simulink model "gm_tutorial1_1_vnl"  (R2020b)
settings: Solver=FixedStepDiscrete  StartTime=0.0  StopTime=simulation_stop_time  RelTol=1e-3
undefined symbols (not defined in the file or in its folder): sample_time
libraries: simulink x3
settings Model: Creator=yixingli  LastModifiedBy=harsh
settings DataIOCC: LimitDataPoints=on  SaveOutput=off  SignalLogging=off  SaveTime=off
settings OptimizationCC: BlockReduction=off  ConditionallyExecuteInputs=off  DefaultParameterBehavior=Inlined  ExpressionDepthLimit=2147483647  LifeSpan=inf
settings DebuggingCC: AlgebraicLoopMsg=error  UnderspecifiedInitializationDetection=Classic  MergeDetectMultiDrivingBlocksExec=none  InheritedTsInSrcMsg=none  SingleTaskRateTransMsg=error  ParameterPrecisionLossMsg=none  AllowSymbolicDim=off  StateNameClashWarn=warning  StrictBusMsg=ErrorOnBusTreatedAsVector  SFUnexpectedBacktrackingDiag=warning  SFNoUnconditionalDefaultTransitionDiag=warning  SFExecutionAtInitializationDiag=none  ArithmeticOperatorsInVariantConditions=warning
settings HardwareCC: ProdBitPerPointer=32  ProdBitPerSizeT=32  ProdBitPerPtrDiffT=32  ProdLargestAtomicFloat=None  ProdIntDivRoundTo=Undefined  ProdEndianess=Unspecified  ProdWordSize=32  ProdHWDeviceType=ASIC/FPGA->ASIC/FPGA  ProdEqTarget=off
settings SFSimCC: SimUseLocalCustomCode=off  CustomCodeUndefinedFunction=UseInterfaceOnly
settings RTWCC: RTWUseLocalCustomCode=off
settings CodeAppCC: StateflowObjectComments=on
settings GRTTargetCC: TargetLangStandard=C89/C90 (ANSI)
settings ConfigComp: CovScope=ReferencedModels  CovMetricSettings=dw  CovSaveCumulativeToWorkspaceVar=on  CovSaveSingleToWorkspaceVar=on  CovExternalEMLEnable=off  CovSFcnEnable=off

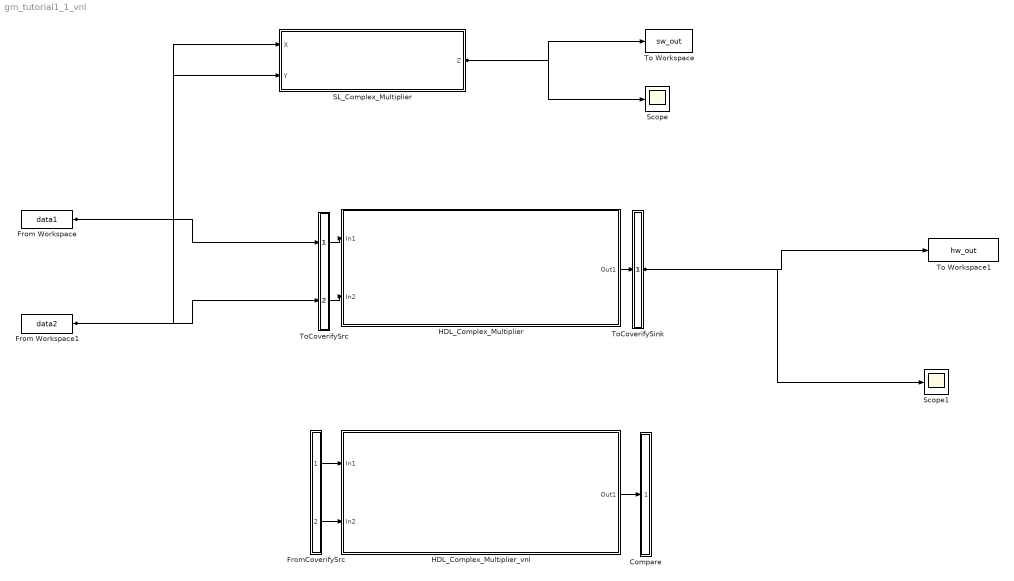
== system gm_tutorial1_1_vnl ==
  Compare : Subsystem
      mask Display: disp('')
  From Workspace : FromWorkspace  VariableName=data1  SampleTime=sample_time  Interpolate=off  OutputAfterFinalValue=Setting to zero
  From Workspace1 : FromWorkspace  VariableName=data2  SampleTime=sample_time  Interpolate=off  OutputAfterFinalValue=Setting to zero
  FromCoverifySrc : Subsystem
      mask Display: disp('')
  HDL_Complex_Multiplier : Subsystem
  HDL_Complex_Multiplier_vnl : Subsystem
  SL_Complex_Multiplier : Subsystem
  Scope : Scope
  Scope1 : Scope
  To Workspace : ToWorkspace  VariableName=sw_out  SaveFormat=Structure With Time  SampleTime=-1
  To Workspace1 : ToWorkspace  VariableName=hw_out  SaveFormat=Structure With Time  SampleTime=-1
  ToCoverifySink : Subsystem
      mask Display: disp('')
  ToCoverifySrc : Subsystem
      mask Display: disp('')
  wires:
  SL_Complex_Multiplier/1(Z) -> To Workspace/1, Scope/1
  From Workspace/1 -> SL_Complex_Multiplier/1(X), ToCoverifySrc/1(in1)
  From Workspace1/1 -> SL_Complex_Multiplier/2(Y), ToCoverifySrc/2(in2)
  ToCoverifySrc/1(out1) -> HDL_Complex_Multiplier/1(In1)
  ToCoverifySrc/2(out2) -> HDL_Complex_Multiplier/2(In2)
  HDL_Complex_Multiplier/1(Out1) -> ToCoverifySink/1(in1)
  ToCoverifySink/1(out1) -> To Workspace1/1, Scope1/1
  FromCoverifySrc/1(out1) -> HDL_Complex_Multiplier_vnl/1(In1)
  FromCoverifySrc/2(out2) -> HDL_Complex_Multiplier_vnl/2(In2)
  HDL_Complex_Multiplier_vnl/1(Out1) -> Compare/1(in1)

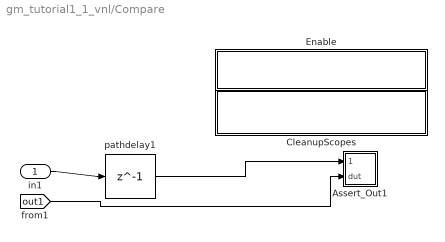
== system gm_tutorial1_1_vnl/Compare ==
  in1 : Inport
  Assert_Out1 : Subsystem
  CleanupScopes : Subsystem
      settings: OpenFcn=|
      | blkName = gcb; %self block
      | idx = regexp(blkName, '/CleanupScopes$', 'once');
      | blkParent = blkName(1:idx-1);
      | blks=find_system(blkParent, 'LookUnderMasks', 'all','blocktype', 'Scope');
      | for itr = 1:length(blks)
      | 	 hScopeCfg = get_param(blks{itr},'ScopeConfiguration');
      | 	 hScopeCfg.Visible = ~ hScopeCfg.Visible;
      | end
      | drawnow;
      mask Display: fprintf(message('hdlcoder:cosim:vnl_dblclick').getString());
  Enable : Subsystem
      settings: OpenFcn=|
      | blkName = gcb;
      | idx = regexp(blkName, '/Enable$', 'once');
      | blkParent = blkName(1:idx-1);
      | blks=find_system(blkParent, 'LookUnderMasks', 'all','blocktype', 'Assertion');
      | e = get_param(blks{1}, 'Enabled');
      | if strcmp(e, 'on'), f= 'off';, else, f = 'on';, end
      | for ii=1:length(blks), set_param(blks{ii}, 'Enabled', f);, end
      | set_param(gcb, 'MaskDisplay',['fprintf(message(''hdlcoder:cosim:vnl_dblclick_assertions'',','''',upper(e),'''',').getString())']);
      mask Display: fprintf(message('hdlcoder:cosim:vnl_dblclick_assertions','OFF').getString());
  pathdelay1 : Delay  DelayLength=1
  wires:
  in1/1 -> pathdelay1/1
  pathdelay1/1 -> Assert_Out1/1(cosim)
  [out1] -> Assert_Out1/2(dut)

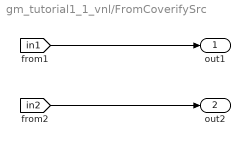
== system gm_tutorial1_1_vnl/FromCoverifySrc ==
  out1 : Outport
  out2 : Outport  Port=2
  wires:
  [in1] -> out1/1
  [in2] -> out2/1

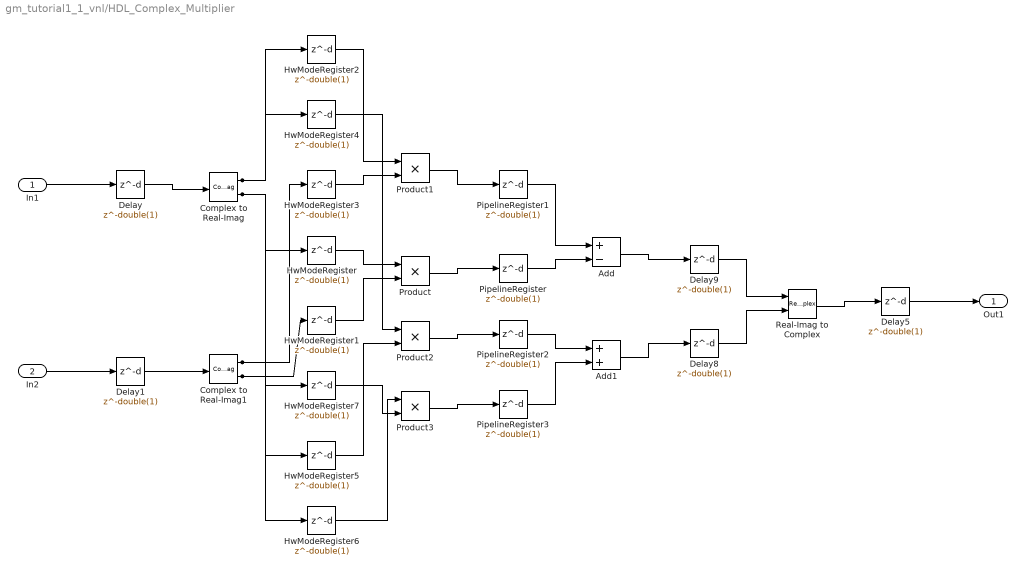
== system gm_tutorial1_1_vnl/HDL_Complex_Multiplier ==
  In1 : Inport  OutDataTypeStr=fixdt(1, 12, 8)  PortDimensions=1  SampleTime=1e-06
      settings: SignalType=complex
  In2 : Inport  Port=2  OutDataTypeStr=fixdt(1, 12, 8)  PortDimensions=1  SampleTime=1e-06
      settings: SignalType=complex
  Add : Sum  Inputs=+-  AccumDataTypeStr=fixdt(1, 25, 16)  OutDataTypeStr=fixdt(1, 25, 16)  SampleTime=1e-06
  Add1 : Sum  AccumDataTypeStr=fixdt(1, 25, 16)  OutDataTypeStr=fixdt(1, 25, 16)  SampleTime=1e-06
  Complex to Real-Imag : ComplexToRealImag  SampleTime=1e-06
  Complex to Real-Imag1 : ComplexToRealImag  SampleTime=1e-06
  Delay{,1,5,8..9} (5 alike) : Delay  DelayLength=double(1)  InitialCondition=0  SampleTime=1e-06
  HwModeRegister{,1..7} (8 alike) : Delay  DelayLength=double(1)  InitialCondition=0  SampleTime=1e-06
  PipelineRegister{,1..3} (4 alike) : Delay  DelayLength=double(1)  InitialCondition=0  SampleTime=1e-06
  Product{,1..3} (4 alike) : Product  Inputs=**  OutDataTypeStr=fixdt(1, 24, 16)  SampleTime=1e-06
  Real-Imag to Complex : RealImagToComplex  ConstantPart="fi(0,1,25,16,\"hex\",\"0000000\")"  SampleTime=1e-06
  Out1 : Outport
  wires:
  HwModeRegister7/1 -> Product3/2
  HwModeRegister6/1 -> Product3/1
  Product3/1 -> PipelineRegister3/1
  HwModeRegister5/1 -> Product2/2
  HwModeRegister4/1 -> Product2/1
  Product2/1 -> PipelineRegister2/1
  HwModeRegister3/1 -> Product1/2
  HwModeRegister2/1 -> Product1/1
  Product1/1 -> PipelineRegister1/1
  HwModeRegister1/1 -> Product/2
  HwModeRegister/1 -> Product/1
  Product/1 -> PipelineRegister/1
  Real-Imag to Complex/1 -> Delay5/1
  PipelineRegister3/1 -> Add1/2
  PipelineRegister2/1 -> Add1/1
  PipelineRegister1/1 -> Add/1
  PipelineRegister/1 -> Add/2
  Delay9/1 -> Real-Imag to Complex/1
  Delay8/1 -> Real-Imag to Complex/2
  Delay5/1 -> Out1/1
  Delay1/1 -> Complex to Real-Imag1/1
  Delay/1 -> Complex to Real-Imag/1
  Complex to Real-Imag1/2 -> HwModeRegister5/1, HwModeRegister1/1
  Complex to Real-Imag1/1 -> HwModeRegister6/1, HwModeRegister3/1
  Complex to Real-Imag/2 -> HwModeRegister7/1, HwModeRegister/1
  Complex to Real-Imag/1 -> HwModeRegister4/1, HwModeRegister2/1
  Add1/1 -> Delay8/1
  Add/1 -> Delay9/1
  In2/1 -> Delay1/1
  In1/1 -> Delay/1

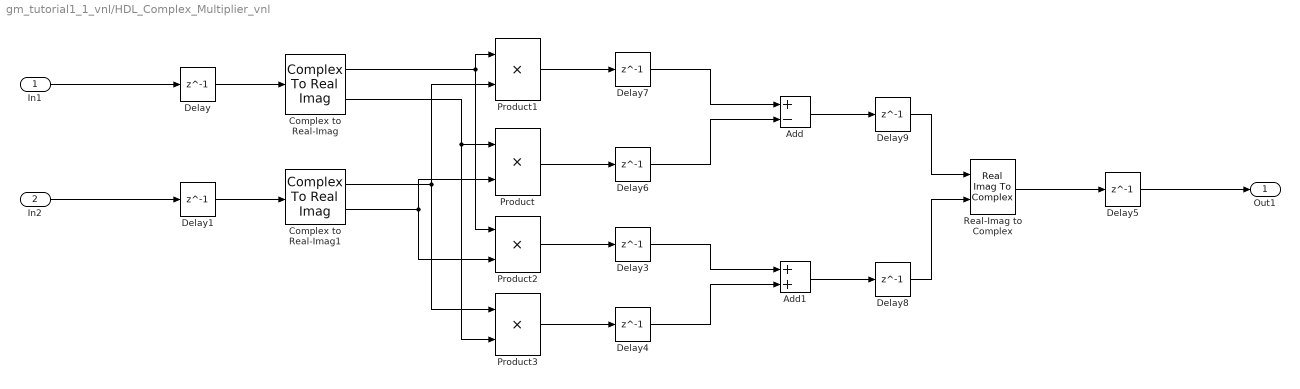
== system gm_tutorial1_1_vnl/HDL_Complex_Multiplier_vnl ==
  In1 : Inport
  In2 : Inport  Port=2
  Add : Sum  Inputs=+-
  Add1 : Sum
  Complex to Real-Imag : ComplexToRealImag
  Complex to Real-Imag1 : ComplexToRealImag
  Delay{,1,3..9} (9 alike) : Delay  DelayLength=1  InitialCondition=0
  Product{,1..3} (4 alike) : Product
  Real-Imag to Complex : RealImagToComplex
  Out1 : Outport
  wires:
  Product1/1 -> Delay7/1
  Delay4/1 -> Add1/2
  Product3/1 -> Delay4/1
  Add1/1 -> Delay8/1
  Add/1 -> Delay9/1
  Product2/1 -> Delay3/1
  Delay5/1 -> Out1/1
  Real-Imag to Complex/1 -> Delay5/1
  In1/1 -> Delay/1
  Complex to Real-Imag1/2 -> Product2/2, Product/2
  Product/1 -> Delay6/1
  In2/1 -> Delay1/1
  Delay/1 -> Complex to Real-Imag/1
  Delay3/1 -> Add1/1
  Complex to Real-Imag/1 -> Product1/1, Product2/1
  Delay6/1 -> Add/2
  Delay7/1 -> Add/1
  Delay8/1 -> Real-Imag to Complex/2
  Delay9/1 -> Real-Imag to Complex/1
  Delay1/1 -> Complex to Real-Imag1/1
  Complex to Real-Imag1/1 -> Product1/2, Product3/1
  Complex to Real-Imag/2 -> Product3/2, Product/1

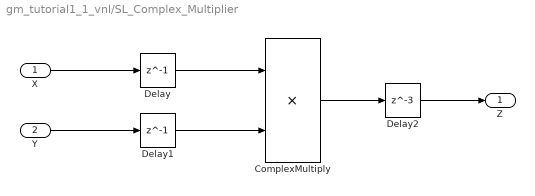
== system gm_tutorial1_1_vnl/SL_Complex_Multiplier ==
  X : Inport
  Y : Inport  Port=2
  ComplexMultiply : Product
  Delay : Delay  DelayLength=1  InitialCondition=0
  Delay1 : Delay  DelayLength=1  InitialCondition=0
  Delay2 : Delay  DelayLength=3  InitialCondition=0
  Z : Outport  VectorParamsAs1DForOutWhenUnconnected=off
  wires:
  ComplexMultiply/1 -> Delay2/1
  X/1 -> Delay/1
  Y/1 -> Delay1/1
  Delay1/1 -> ComplexMultiply/2
  Delay/1 -> ComplexMultiply/1
  Delay2/1 -> Z/1

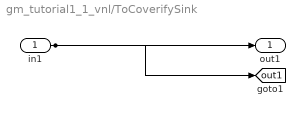
== system gm_tutorial1_1_vnl/ToCoverifySink ==
  in1 : Inport
  out1 : Outport
  tag scope: out1=global
  wires:
  in1/1 -> out1/1, [out1]

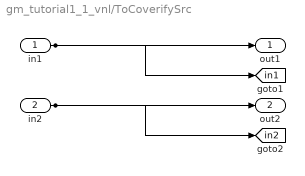
== system gm_tutorial1_1_vnl/ToCoverifySrc ==
  in1 : Inport
  in2 : Inport  Port=2
  out1 : Outport
  out2 : Outport  Port=2
  tag scope: in1=global, in2=global
  wires:
  in1/1 -> out1/1, [in1]
  in2/1 -> out2/1, [in2]

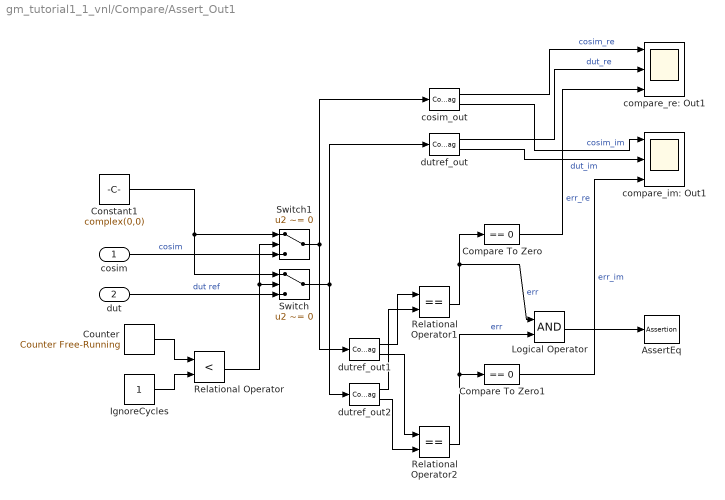
== system gm_tutorial1_1_vnl/Compare/Assert_Out1 ==
  cosim : Inport
  dut : Inport  Port=2
  AssertEq : Assertion  StopWhenAssertionFail=off
  Compare To Zero : simulink/Logic and Bit Operations/Compare To Zero  relop===  OutDataTypeStr=boolean
  Compare To Zero1 : simulink/Logic and Bit Operations/Compare To Zero  relop===  OutDataTypeStr=boolean
  Constant1 : Constant  Value=complex(0,0)  OutDataTypeStr=Inherit: Inherit via back propagation  SampleTime=-1
  Counter : simulink/Sources/Counter Free-Running  NumBits=32  tsamp=-1
  IgnoreCycles : Constant  OutDataTypeStr=Inherit: Inherit via back propagation  SampleTime=-1
  Logical Operator : Logic  AllPortsSameDT=off  OutDataTypeStr=boolean
  Relational Operator : RelationalOperator  Operator=<  OutDataTypeStr=boolean  RndMeth=Nearest
  Relational Operator1 : RelationalOperator  Operator===  OutDataTypeStr=boolean  RndMeth=Nearest
  Relational Operator2 : RelationalOperator  Operator===  OutDataTypeStr=boolean  RndMeth=Nearest
  Switch : Switch  Criteria=u2 ~= 0
  Switch1 : Switch  Criteria=u2 ~= 0
  compare_im: Out1 : Scope  NumInputPorts=3
  compare_re: Out1 : Scope  NumInputPorts=3
  cosim_out : ComplexToRealImag
  dutref_out : ComplexToRealImag
  dutref_out1 : ComplexToRealImag
  dutref_out2 : ComplexToRealImag
  wires:
  Relational Operator2/1 -> Compare To Zero1/1, Logical Operator/2  "err"
  dutref_out1/2 -> Relational Operator2/1
  dutref_out2/2 -> Relational Operator2/2
  dutref_out2/1 -> Relational Operator1/2
  dutref_out1/1 -> Relational Operator1/1
  Logical Operator/1 -> AssertEq/1
  IgnoreCycles/1 -> Relational Operator/2
  Counter/1 -> Relational Operator/1
  dut/1 -> Switch/3  "dut ref"
  cosim/1 -> Switch1/3  "cosim"
  Relational Operator/1 -> Switch/2, Switch1/2
  Constant1/1 -> Switch/1, Switch1/1
  Switch/1 -> dutref_out/1, dutref_out2/1
  Switch1/1 -> cosim_out/1, dutref_out1/1
  Relational Operator1/1 -> Compare To Zero/1, Logical Operator/1  "err"
  cosim_out/1 -> compare_re: Out1/1  "cosim_re"
  dutref_out/1 -> compare_re: Out1/2  "dut_re"
  Compare To Zero/1 -> compare_re: Out1/3  "err_re"
  cosim_out/2 -> compare_im: Out1/1  "cosim_im"
  dutref_out/2 -> compare_im: Out1/2  "dut_im"
  Compare To Zero1/1 -> compare_im: Out1/3  "err_im"

== system gm_tutorial1_1_vnl/Compare/CleanupScopes ==

== system gm_tutorial1_1_vnl/Compare/Enable ==
